simulink model "model1b"  (R2014b)
settings: Solver=ode45  StartTime=0.0  StopTime=20.0  RelTol=1e-3
settings Model: Creator=Shane Reynolds  LastModifiedBy=Shane Reynolds

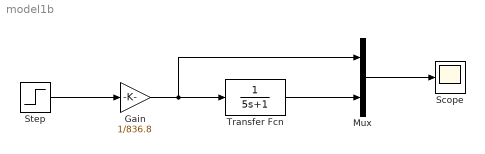
== system model1b ==
  Gain : Gain  Gain=1/836.8
  Mux : Mux  Inputs=2
  Scope : Scope
  Step : Step  After=2520  SampleTime=0
  Transfer Fcn : TransferFcn  Denominator=[5 1]
  wires:
  Step/1 -> Gain/1
  Gain/1 -> Mux/1, Transfer Fcn/1
  Transfer Fcn/1 -> Mux/2
  Mux/1 -> Scope/1
